simulink model "realvleospacecraft0LB_mpcpd"  (R2022b)
settings: Solver=VariableStepAuto  StartTime=0.0  StopTime=200  MaxStep=1  RelTol=1e-3  AbsTol=1e-3
StopFcn:
  | sim_complete = true;
undefined symbols (not defined in the file or in its folder): cont_update, costfunction, mpcpd, tar
settings Model: Creator=Abhijit  LastModifiedBy=abhij
settings SolverCC: AutoScaleAbsTol=off  AlgebraicLoopSolver=TrustRegion  MaxZcPerStep=1
settings DataIOCC: SaveOperatingPoint=on  SaveState=on  StateSaveName=states
settings DebuggingCC: UnconnectedInputMsg=warning  UnconnectedOutputMsg=warning  UnconnectedLineMsg=warning  SymbolicDimsDataTypeCodeGenerationDiagnostic=none  SFMachineParentedDataDiag=warning
settings ModelReferenceCC: EnableRefExpFcnMdlSchedulingChecks=on
settings SFSimCC: CustomCodeUndefinedFunction=UseInterfaceOnly
settings RTWCC: DLArmComputeVersion=19.05
settings SimscapeCC: SimscapeLogType=all  SimscapeLogSimulationStatistics=on  SimscapeLogDataHistory=10000

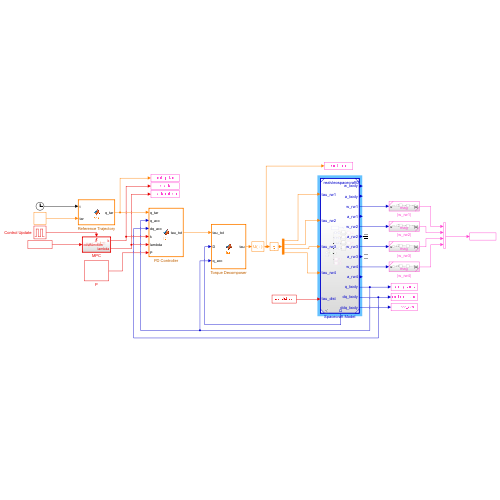
[thumbnail: Simulink's stored preview of the top-level diagram]
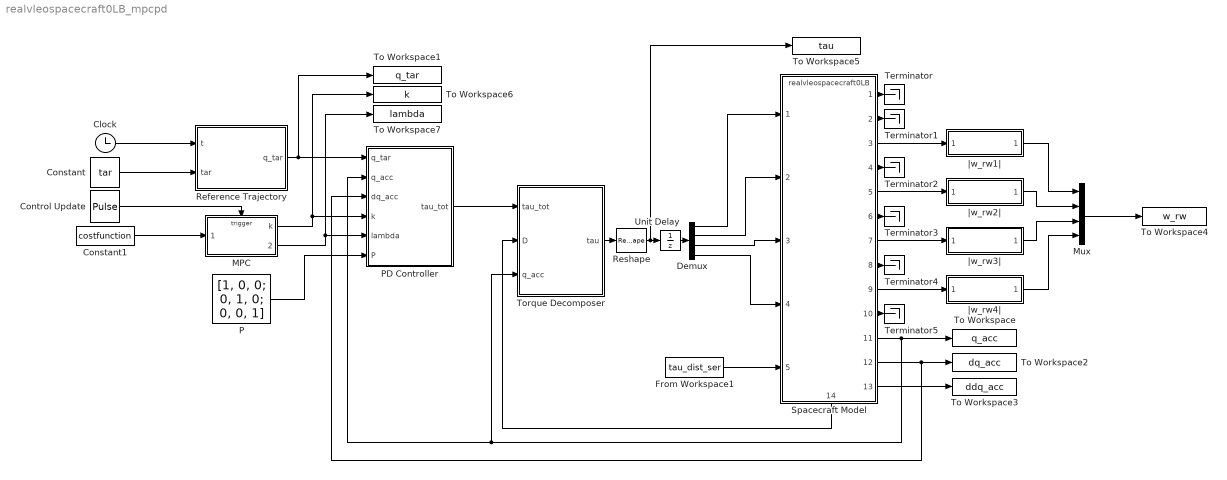
== system realvleospacecraft0LB_mpcpd ==
  Clock : Clock
  Constant : Constant  Value=tar
  Constant1 : Constant  Value=costfunction
  Control Update : DiscretePulseGenerator  PulseType=Time based  Period=cont_update  PulseWidth=5  PhaseDelay=0.1
  Demux : Demux
  From Workspace1 : FromWorkspace  VariableName=tau_dist_ser  Interpolate=off  OutputAfterFinalValue=Holding final value
  MPC : Subsystem
  Mux : Mux
  P : Constant  Value=[1, 0, 0; 0, 1, 0; 0, 0, 1]
  PD Controller : MATLAB Function  TreatAsAtomicUnit=on
  Reference Trajectory : MATLAB Function  TreatAsAtomicUnit=on
  Reshape : Reshape
  Spacecraft Model : ModelReference  ModelNameDialog=realvleospacecraft0LB  SimulationMode=Normal  ModelReferenceVersion=1.30
      settings: PortSchema="{\"entries\":[{\"content\":{\"sides\":[{\"content\":{\"connectorIds\":[\"In1\",\"In2\",\"In3\",\"In4\",\"In5\"]},\"type\":\"ConnectorPlacement.EquallySpacedRectSide\",\"uuid\":\"36a9c944-f213-4c4e-b6f2-fa7d728627b0\"},{\"content\":{\"connectorIds\":[\"Out1\",\"Out2\",\"Out3\",\"Out4\",\"Out5\",\"Out6\",\"Out7\",\"Out8\",\"Out9\",\"Out10\",\"Out11\",\"Out12\",\"Out13\"],\"side\":\"RIGHT\"},\"type\":\"ConnectorPlacement.EquallySpacedRectSide\",\"uuid\":\"ad793041-f32f-405f-9966-9455be290c1c\"},{\"content\":{\"connectorIds\":[],\"side\":\"TOP\"},\"type\":\"ConnectorPlacement.EquallySpacedRectSide\",\"uuid\":\"a8d37d27-2c3a-480b-9200-d310321df053\"},{\"content\":{\"connectorIds\":[\"Out14\"],\"side\":\"BOTTOM\"},\"type\":\"ConnectorPlacement.EquallySpacedRectSide\",\"uuid\":\"42546c36-6810-4b9b-bafe-a7a09e10a567\"}]},\"type\":\"ConnectorPlacement.EquallySpacedConnector\",\"uuid\":\"5842ca05-faf4-4c84-934b-15246120a6a0\"}],\"packageUris\":[\"http://schema.mathworks.com/mf0/Connector/R2020b\"],\"version\":\"1.0\"}"
  Terminator{,1..5} (6 alike) : Terminator
  To Workspace : ToWorkspace  VariableName=q_acc  SaveFormat=Timeseries  SampleTime=-1
  To Workspace1 : ToWorkspace  VariableName=q_tar  SaveFormat=Timeseries  SampleTime=-1
  To Workspace2 : ToWorkspace  VariableName=dq_acc  SaveFormat=Timeseries  SampleTime=-1
  To Workspace3 : ToWorkspace  VariableName=ddq_acc  SaveFormat=Timeseries  SampleTime=-1
  To Workspace4 : ToWorkspace  VariableName=w_rw  SaveFormat=Timeseries  SampleTime=-1
  To Workspace5 : ToWorkspace  VariableName=tau  SaveFormat=Timeseries  SampleTime=-1
  To Workspace6 : ToWorkspace  VariableName=k  SaveFormat=Timeseries  SampleTime=-1
  To Workspace7 : ToWorkspace  VariableName=lambda  SaveFormat=Timeseries  SampleTime=-1
  Torque Decomposer : MATLAB Function  TreatAsAtomicUnit=on
  Unit Delay : UnitDelay  SampleTime=-1  HasFrameUpgradeWarning=on
  |w_rw1| : Subsystem  ReferencedSubsystem=mag
  |w_rw2| : Subsystem  ReferencedSubsystem=mag
  |w_rw3| : Subsystem  ReferencedSubsystem=mag
  |w_rw4| : Subsystem  ReferencedSubsystem=mag
  wires:
  Clock/1 -> Reference Trajectory/1(t)
  P/1 -> PD Controller/6(P)
  Reference Trajectory/1(q_tar) -> PD Controller/1(q_tar), To Workspace1/1
  |w_rw3|/1 -> Mux/3
  Spacecraft Model/5 -> |w_rw2|/1
  |w_rw1|/1 -> Mux/1
  Spacecraft Model/12 -> To Workspace2/1, PD Controller/3(dq_acc)
  Spacecraft Model/9 -> |w_rw4|/1
  Demux/2 -> Spacecraft Model/2
  Spacecraft Model/7 -> |w_rw3|/1
  Spacecraft Model/3 -> |w_rw1|/1
  |w_rw4|/1 -> Mux/4
  Demux/3 -> Spacecraft Model/3
  Spacecraft Model/13 -> To Workspace3/1
  Demux/4 -> Spacecraft Model/4
  Demux/1 -> Spacecraft Model/1
  Spacecraft Model/14 -> Torque Decomposer/2(D)
  |w_rw2|/1 -> Mux/2
  Spacecraft Model/11 -> To Workspace/1, PD Controller/2(q_acc), Torque Decomposer/3(q_acc)
  PD Controller/1(tau_tot) -> Torque Decomposer/1(tau_tot)
  Control Update/1 -> MPC/Trigger
  MPC/2(lambda) -> To Workspace7/1, PD Controller/5(lambda)
  MPC/1(k) -> PD Controller/4(k), To Workspace6/1
  Mux/1 -> To Workspace4/1
  Constant/1 -> Reference Trajectory/2(tar)
  Constant1/1 -> MPC/1(costfunction)
  Spacecraft Model/1 -> Terminator/1
  Spacecraft Model/2 -> Terminator1/1
  Spacecraft Model/4 -> Terminator2/1
  Spacecraft Model/6 -> Terminator3/1
  Spacecraft Model/8 -> Terminator4/1
  Spacecraft Model/10 -> Terminator5/1
  Unit Delay/1 -> Demux/1
  Torque Decomposer/1(tau) -> Reshape/1
  Reshape/1 -> To Workspace5/1, Unit Delay/1
  From Workspace1/1 -> Spacecraft Model/5

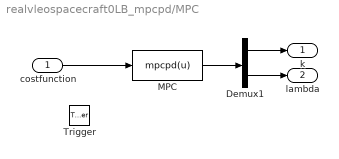
== system realvleospacecraft0LB_mpcpd/MPC ==
  costfunction : Inport
  Trigger : TriggerPort  VariantControl=(inherit)  PortDimensions=1
  Demux1 : Demux  Outputs=2
  MPC : MATLABFcn  MATLABFcn=mpcpd(u)  OutputDimensions=6
  k : Outport
  lambda : Outport  Port=2
  wires:
  Demux1/1 -> k/1
  Demux1/2 -> lambda/1
  MPC/1 -> Demux1/1
  costfunction/1 -> MPC/1

== matlab function realvleospacecraft0LB_mpcpd/PD Controller ==
  data: tau_tot output; q_tar input; q_acc input; dq_acc input; k input; lambda input; P input
function tau_tot = fcn(q_tar, q_acc, dq_acc, k, lambda, P)
    tau_tot = pdcontroller(q_tar, q_acc, dq_acc, k, lambda, P);
end

== matlab function realvleospacecraft0LB_mpcpd/Reference Trajectory ==
  settings: updateMethod=CONTINUOUS
  data: t input; q_tar output; tar input
function q_tar = fcn(t, tar)
     q_tar = refpath(t, tar);
end

== matlab function realvleospacecraft0LB_mpcpd/Torque Decomposer ==
  data: tau_tot input; tau output; D input; q_acc input
function tau = fcn(tau_tot, D, q_acc)
    tau = taudecomp(tau_tot, D, q_acc);
end
